simulink model "state_control_last_model"  (R2024a)
settings: Solver=VariableStepAuto  StartTime=0.0  StopTime=10.0  RelTol=1e-3
values from neighbouring files (symbols this model uses):
  A = [-1.7, -0.25, 0 ... (first row only)    [main.m]
  B = [7, 0 ... (first row only)    [main.m]
  C = [0, 1, 0 ... (first row only)    [main.m]
  x0 = [1 100 200]'    [main.m]
settings Model: Creator=chint  LastModifiedBy=chint

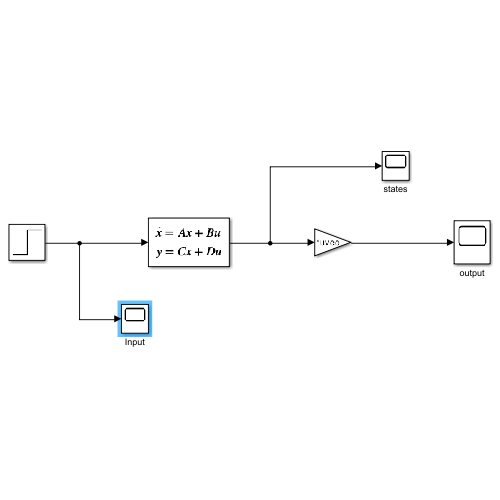
[thumbnail: Simulink's stored preview of the top-level diagram]
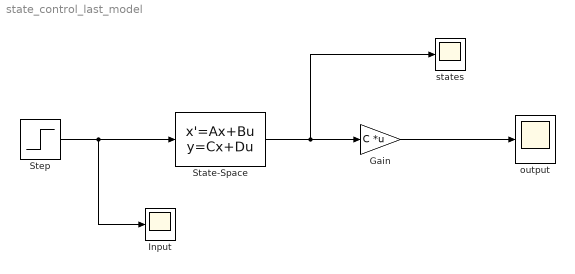
== system state_control_last_model ==
  Gain : Gain  Gain=C  Multiplication=Matrix(K*u) (u vector)
  Input : Scope
  State-Space : StateSpace  A=A  B=B  C=eye(3)  D=zeros(3,2)  InitialCondition=x0
  Step : Step  Before=[0;0]  After=u  SampleTime=0
  output : Scope
  states : Scope
  wires:
  Step/1 -> Input/1, State-Space/1
  State-Space/1 -> states/1, Gain/1
  Gain/1 -> output/1
